simulink model "adas_acc_simulink"  (Simulink 8.8)
settings: Solver=FixedStepDiscrete  StartTime=0.0  StopTime=inf  RelTol=1e-3  EnableMultiTasking=on
libraries: SCANeR_API x7, simulink x3
settings Model: Creator=Administrateur  LastModifiedBy=gadam
settings OptimizationCC: ExpressionDepthLimit=2147483647  InitFltsAndDblsToZero=on  LifeSpan=1
settings DebuggingCC: SolverPrmCheckMsg=warning
settings SFSimCC: SimParseCustomCode=off
settings RTWCC: SystemTargetFile=ert_scanerapi.tlc  TemplateMakefile=ert_scanerapi_vc.tmf  Description=SCANeR API Real-Time Workshop Embedded Coder (no auto configuration)  TargetLang=C++
settings CodeAppCC: IgnoreCustomStorageClasses=off  CustomSymbolStrType=$N$R$M  InternalIdentifier=Classic
settings STFCustomTargetCC: ModelReferenceCompliant=off  CombineOutputUpdateFcns=on  ERTCustomFileBanners=on  RemoveResetFunc=on  MATLABClassNameForMDSCustomization=Simulink.SoftwareTarget.ERTCustomization  CPPClassGenCompliant=on  GRTInterface=off  SystemTargetFile=ert_scanerapi.tlc
settings ERTTargetCC: MultiwordLength=2048  ModelReferenceCompliant=off  ParMdlRefBuildCompliant=off  CompOptLevelCompliant=off  ConcurrentExecutionCompliant=off  ERTFirstTimeCompliant=off  SupportContinuousTime=on  SupportNonInlinedSFcns=on  ModelStepFunctionPrototypeControlCompliant=off  UseToolchainInfoCompliant=off  ExtModeMexFile=noextcomm  ERTCustomFileTemplate=example_file_process.tlc  ConvertIfToSwitch=off  SuppressUnreachableDefaultCases=off
settings CustomProperty: DataType=string  Value=M:\SCANER~1.4\APIs\simulink\SCANER~1

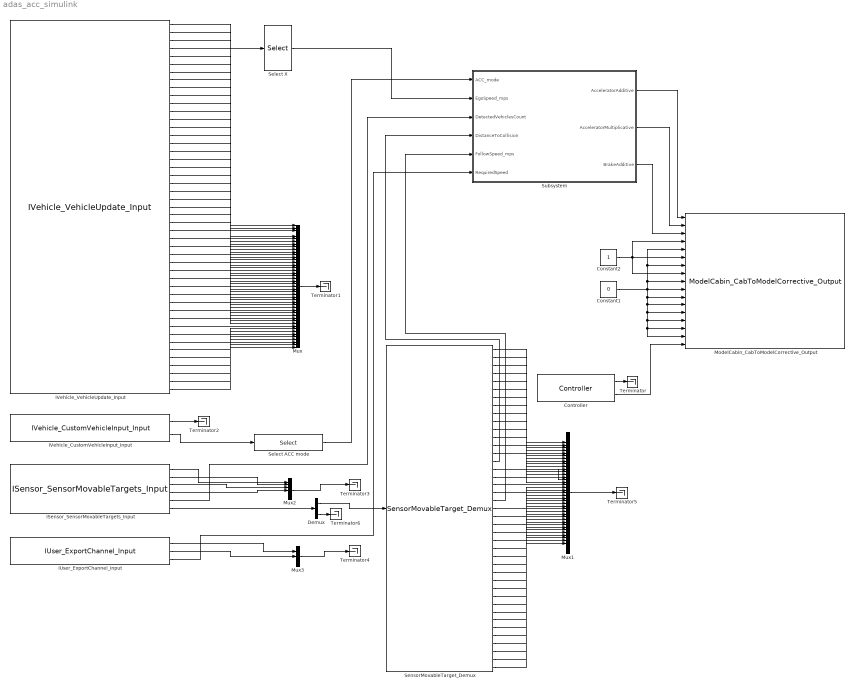
== system adas_acc_simulink ==
  Constant1 : Constant  Value=0
  Constant2 : Constant
  Controller : SCANeR_API/Controller  Config='DEMO_ADAS'  ProcName='SIMULINK_ACC'  Frequency=100  NetworkOutputFrequency=10  TimeOut=30  IsSynchronized=off
  Demux : Demux  Outputs=2
  ISensor_SensorMovableTargets_Input : SCANeR_API/Network inputs/ISensor/ISensor_SensorMovableTargets_Input  Priority=2  ev=off  globalId=300000
  IUser_ExportChannel_Input : SCANeR_API/Network inputs/IUser/IUser_ExportChannel_Input  Priority=2  ev=off  no=66
  IVehicle_CustomVehicleInput_Input : SCANeR_API/Network inputs/IVehicle/IVehicle_CustomVehicleInput_Input  Priority=2  ev=off  vhlId=0
  IVehicle_VehicleUpdate_Input : SCANeR_API/Network inputs/IVehicle/IVehicle_VehicleUpdate_Input  Priority=2  ev=off  vhlId=0
  ModelCabin_CabToModelCorrective_Output : SCANeR_API/SHM outputs/ModelCabin/ModelCabin_CabToModelCorrective_Output  Priority=2  shmId=0
  Mux : Mux  Inputs=47
  Mux1 : Mux  Inputs=39
  Mux2 : Mux  Inputs=6
  Mux3 : Mux  Inputs=3
  Select ACC mode : Selector  IndexMode=Zero-based  InputPortWidth=256  IndexOptions=Index vector (dialog)  Indices=2  OutputSizes=1
  Select X : Selector  IndexMode=Zero-based  InputPortWidth=6  IndexOptions=Index vector (dialog)  Indices=0  OutputSizes=1
  SensorMovableTarget_Demux : SCANeR_API/Structures/SensorMovableTarget_Demux
  Subsystem : Subsystem
  Terminator{,1..6} (7 alike) : Terminator
  wires:
  Controller/2 -> ModelCabin_CabToModelCorrective_Output/17
  Controller/1 -> Terminator/1
  Constant1/1 -> ModelCabin_CabToModelCorrective_Output/5, ModelCabin_CabToModelCorrective_Output/7, ModelCabin_CabToModelCorrective_Output/9, ModelCabin_CabToModelCorrective_Output/11, ModelCabin_CabToModelCorrective_Output/12, ModelCabin_CabToModelCorrective_Output/13, ModelCabin_CabToModelCorrective_Output/14, ModelCabin_CabToModelCorrective_Output/15, ModelCabin_CabToModelCorrective_Output/16, ModelCabin_CabToModelCorrective_Output/10
  Constant2/1 -> ModelCabin_CabToModelCorrective_Output/4, ModelCabin_CabToModelCorrective_Output/6, ModelCabin_CabToModelCorrective_Output/8
  IVehicle_VehicleUpdate_Input/39 -> Mux/39
  IVehicle_VehicleUpdate_Input/38 -> Mux/38
  IVehicle_VehicleUpdate_Input/40 -> Mux/40
  IVehicle_VehicleUpdate_Input/37 -> Mux/37
  IVehicle_VehicleUpdate_Input/41 -> Mux/41
  IVehicle_VehicleUpdate_Input/36 -> Mux/36
  IVehicle_VehicleUpdate_Input/42 -> Mux/42
  IVehicle_VehicleUpdate_Input/35 -> Mux/35
  IVehicle_VehicleUpdate_Input/43 -> Mux/43
  IVehicle_VehicleUpdate_Input/34 -> Mux/34
  IVehicle_VehicleUpdate_Input/44 -> Mux/44
  IVehicle_VehicleUpdate_Input/33 -> Mux/33
  IVehicle_VehicleUpdate_Input/45 -> Mux/45
  IVehicle_VehicleUpdate_Input/32 -> Mux/32
  IVehicle_VehicleUpdate_Input/46 -> Mux/46
  IVehicle_VehicleUpdate_Input/31 -> Mux/31
  IVehicle_VehicleUpdate_Input/47 -> Mux/47
  IVehicle_VehicleUpdate_Input/30 -> Mux/30
  IVehicle_VehicleUpdate_Input/29 -> Mux/29
  IVehicle_VehicleUpdate_Input/28 -> Mux/28
  IVehicle_VehicleUpdate_Input/27 -> Mux/27
  IVehicle_VehicleUpdate_Input/26 -> Mux/26
  IVehicle_VehicleUpdate_Input/25 -> Mux/25
  IVehicle_VehicleUpdate_Input/24 -> Mux/24
  IVehicle_VehicleUpdate_Input/23 -> Mux/23
  IVehicle_VehicleUpdate_Input/22 -> Mux/22
  IVehicle_VehicleUpdate_Input/21 -> Mux/21
  IVehicle_VehicleUpdate_Input/20 -> Mux/20
  IVehicle_VehicleUpdate_Input/19 -> Mux/19
  IVehicle_VehicleUpdate_Input/18 -> Mux/18
  IVehicle_VehicleUpdate_Input/17 -> Mux/17
  IVehicle_VehicleUpdate_Input/16 -> Mux/16
  IVehicle_VehicleUpdate_Input/15 -> Mux/15
  IVehicle_VehicleUpdate_Input/14 -> Mux/14
  IVehicle_VehicleUpdate_Input/13 -> Mux/13
  IVehicle_VehicleUpdate_Input/12 -> Mux/12
  IVehicle_VehicleUpdate_Input/11 -> Mux/11
  IVehicle_VehicleUpdate_Input/10 -> Mux/10
  IVehicle_VehicleUpdate_Input/9 -> Mux/9
  IVehicle_VehicleUpdate_Input/8 -> Mux/8
  IVehicle_VehicleUpdate_Input/7 -> Mux/7
  IVehicle_VehicleUpdate_Input/6 -> Mux/6
  IVehicle_VehicleUpdate_Input/5 -> Mux/5
  IVehicle_VehicleUpdate_Input/3 -> Mux/3
  IVehicle_VehicleUpdate_Input/2 -> Mux/2
  IVehicle_VehicleUpdate_Input/1 -> Mux/1
  ISensor_SensorMovableTargets_Input/3 -> Mux2/3
  ISensor_SensorMovableTargets_Input/4 -> Mux2/4
  ISensor_SensorMovableTargets_Input/2 -> Mux2/2
  ISensor_SensorMovableTargets_Input/1 -> Mux2/1
  IUser_ExportChannel_Input/2 -> Mux3/2
  IUser_ExportChannel_Input/1 -> Mux3/1
  Mux3/1 -> Terminator4/1
  Mux2/1 -> Terminator3/1
  Mux/1 -> Terminator1/1
  Subsystem/3(BrakeAdditive) -> ModelCabin_CabToModelCorrective_Output/3
  Subsystem/2(AcceleratorMultiplicative) -> ModelCabin_CabToModelCorrective_Output/2
  Subsystem/1(AcceleratorAdditive) -> ModelCabin_CabToModelCorrective_Output/1
  IVehicle_CustomVehicleInput_Input/1 -> Terminator2/1
  IVehicle_VehicleUpdate_Input/4 -> Select X/1
  Select X/1 -> Subsystem/2(EgoSpeed_mps)
  ISensor_SensorMovableTargets_Input/5 -> Subsystem/3(DetectedVehiclesCount)
  ISensor_SensorMovableTargets_Input/6 -> Demux/1
  Demux/1 -> SensorMovableTarget_Demux/1
  SensorMovableTarget_Demux/15 -> Subsystem/4(DistanceToCollision)
  SensorMovableTarget_Demux/20 -> Subsystem/5(FollowSpeed_mps)
  IUser_ExportChannel_Input/3 -> Subsystem/6(RequiredSpeed)
  SensorMovableTarget_Demux/16 -> Mux1/15
  SensorMovableTarget_Demux/17 -> Mux1/16
  SensorMovableTarget_Demux/18 -> Mux1/17
  SensorMovableTarget_Demux/14 -> Mux1/14
  SensorMovableTarget_Demux/19 -> Mux1/18
  SensorMovableTarget_Demux/13 -> Mux1/13
  SensorMovableTarget_Demux/12 -> Mux1/12
  SensorMovableTarget_Demux/11 -> Mux1/11
  SensorMovableTarget_Demux/21 -> Mux1/19
  SensorMovableTarget_Demux/10 -> Mux1/10
  SensorMovableTarget_Demux/22 -> Mux1/20
  SensorMovableTarget_Demux/9 -> Mux1/9
  SensorMovableTarget_Demux/23 -> Mux1/21
  SensorMovableTarget_Demux/8 -> Mux1/8
  SensorMovableTarget_Demux/24 -> Mux1/22
  SensorMovableTarget_Demux/7 -> Mux1/7
  SensorMovableTarget_Demux/25 -> Mux1/23
  SensorMovableTarget_Demux/6 -> Mux1/6
  SensorMovableTarget_Demux/26 -> Mux1/24
  SensorMovableTarget_Demux/5 -> Mux1/5
  SensorMovableTarget_Demux/27 -> Mux1/25
  SensorMovableTarget_Demux/4 -> Mux1/4
  SensorMovableTarget_Demux/28 -> Mux1/26
  SensorMovableTarget_Demux/3 -> Mux1/3
  SensorMovableTarget_Demux/29 -> Mux1/27
  SensorMovableTarget_Demux/2 -> Mux1/2
  SensorMovableTarget_Demux/30 -> Mux1/28
  SensorMovableTarget_Demux/1 -> Mux1/1
  SensorMovableTarget_Demux/31 -> Mux1/29
  SensorMovableTarget_Demux/32 -> Mux1/30
  SensorMovableTarget_Demux/33 -> Mux1/31
  SensorMovableTarget_Demux/34 -> Mux1/32
  SensorMovableTarget_Demux/35 -> Mux1/33
  SensorMovableTarget_Demux/36 -> Mux1/34
  SensorMovableTarget_Demux/37 -> Mux1/35
  SensorMovableTarget_Demux/38 -> Mux1/36
  SensorMovableTarget_Demux/39 -> Mux1/37
  SensorMovableTarget_Demux/40 -> Mux1/38
  SensorMovableTarget_Demux/41 -> Mux1/39
  Mux1/1 -> Terminator5/1
  Demux/2 -> Terminator6/1
  Select ACC mode/1 -> Subsystem/1(ACC_mode)
  IVehicle_CustomVehicleInput_Input/2 -> Select ACC mode/1

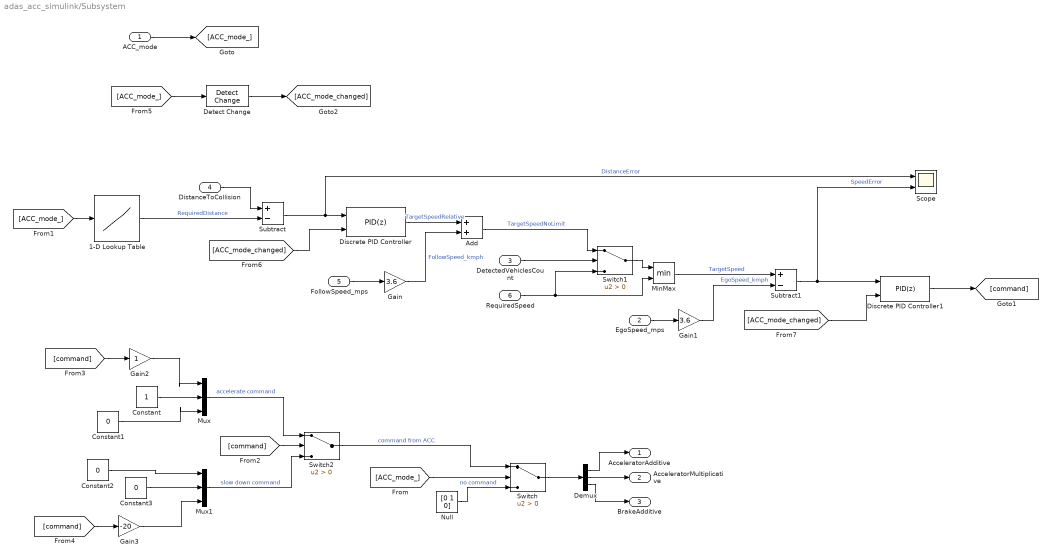
== system adas_acc_simulink/Subsystem ==
  ACC_mode : Inport
  EgoSpeed_mps : Inport  Port=2
  DetectedVehiclesCount : Inport  Port=3
  DistanceToCollision : Inport  Port=4
  FollowSpeed_mps : Inport  Port=5
  RequiredSpeed : Inport  Port=6
  1-D Lookup Table : Lookup_n-D  NumberOfTableDimensions=1  BreakpointsSpecification=Even spacing  BreakpointsForDimension1=[1,2,3,4]  Table=[20,30,40,50]  InternalRulePriority=Speed  RndMeth=Simplest  InputSameDT=on
  Add : Sum
  Constant : Constant
  Constant1 : Constant  Value=0
  Constant2 : Constant  Value=0
  Constant3 : Constant  Value=0
  Demux : Demux  Outputs=3
  Detect Change : simulink/Logic and Bit Operations/Detect Change  vinit=0  OutDataTypeStr=boolean
  Discrete PID Controller : simulink/Continuous/PID Controller  Controller=PID  TimeDomain=Discrete-time  SampleTime=-1  IntegratorMethod=Forward Euler  FilterMethod=Forward Euler  Form=Parallel  UseFilter=on  ControllerParametersSource=internal  P=0.5  I=1e-4  D=0.5  N=100  InitialConditionSource=internal  InitialConditionForIntegrator=0  InitialConditionForFilter=0  ExternalReset=rising  LimitOutput=on  UpperSaturationLimit=200  LowerSaturationLimit=0  LinearizeAsGain=off  AntiWindupMode=none  Kb=1  TrackingMode=off  Kt=1  PParamMin=[]  PParamMax=[]  IParamMin=[]  IParamMax=[]  DParamMin=[]  DParamMax=[]  NParamMin=[]  NParamMax=[]  KbParamMin=[]  KbParamMax=[]  KtParamMin=[]  KtParamMax=[]  POutMin=[]  POutMax=[]  IOutMin=[]  IOutMax=[]  DOutMin=[]  DOutMax=[]  NOutMin=[]  NOutMax=[]  KbOutMin=[]  KbOutMax=[]  KtOutMin=[]  KtOutMax=[]  IntegratorOutMin=[]  IntegratorOutMax=[]  FilterOutMin=[]  FilterOutMax=[]  SumOutMin=[]  SumOutMax=[]  SumI1OutMin=[]  SumI1OutMax=[]  SumI2OutMin=[]  SumI2OutMax=[]  SumI3OutMin=[]  SumI3OutMax=[]  SumDOutMin=[]  SumDOutMax=[]  SaturationOutMin=[]  SaturationOutMax=[]  IntegratorContinuousStateAttributes=''  IntegratorStateMustResolveToSignalObject=off  IntegratorRTWStateStorageClass=Auto  FilterContinuousStateAttributes=''  FilterStateMustResolveToSignalObject=off  FilterRTWStateStorageClass=Auto  DifferentiatorICPrevScaledInput=0  DifferentiatorOutMin=[]  DifferentiatorOutMax=[]
  Discrete PID Controller1 : simulink/Continuous/PID Controller  Controller=PID  TimeDomain=Discrete-time  SampleTime=-1  IntegratorMethod=Forward Euler  FilterMethod=Forward Euler  Form=Parallel  UseFilter=on  ControllerParametersSource=internal  P=0.1  I=5e-4  D=0.1  N=100  InitialConditionSource=internal  InitialConditionForIntegrator=0  InitialConditionForFilter=0  ExternalReset=rising  LimitOutput=on  UpperSaturationLimit=1  LowerSaturationLimit=-1  LinearizeAsGain=off  AntiWindupMode=none  Kb=1  TrackingMode=off  Kt=1  PParamMin=[]  PParamMax=[]  IParamMin=[]  IParamMax=[]  DParamMin=[]  DParamMax=[]  NParamMin=[]  NParamMax=[]  KbParamMin=[]  KbParamMax=[]  KtParamMin=[]  KtParamMax=[]  POutMin=[]  POutMax=[]  IOutMin=[]  IOutMax=[]  DOutMin=[]  DOutMax=[]  NOutMin=[]  NOutMax=[]  KbOutMin=[]  KbOutMax=[]  KtOutMin=[]  KtOutMax=[]  IntegratorOutMin=[]  IntegratorOutMax=[]  FilterOutMin=[]  FilterOutMax=[]  SumOutMin=[]  SumOutMax=[]  SumI1OutMin=[]  SumI1OutMax=[]  SumI2OutMin=[]  SumI2OutMax=[]  SumI3OutMin=[]  SumI3OutMax=[]  SumDOutMin=[]  SumDOutMax=[]  SaturationOutMin=[]  SaturationOutMax=[]  IntegratorContinuousStateAttributes=''  IntegratorStateMustResolveToSignalObject=off  IntegratorRTWStateStorageClass=Auto  FilterContinuousStateAttributes=''  FilterStateMustResolveToSignalObject=off  FilterRTWStateStorageClass=Auto  DifferentiatorICPrevScaledInput=0  DifferentiatorOutMin=[]  DifferentiatorOutMax=[]
  Gain : Gain  Gain=3.6
  Gain1 : Gain  Gain=3.6
  Gain2 : Gain
  Gain3 : Gain  Gain=-20
  MinMax : MinMax  Inputs=2
  Mux : Mux  Inputs=3
  Mux1 : Mux  Inputs=3
  Null : Constant  Value=[0 1 0]
  Scope : Scope  NumInputPorts=2
  Subtract : Sum  Inputs=+-
  Subtract1 : Sum  Inputs=+-
  Switch : Switch  Criteria=u2 > Threshold
  Switch1 : Switch  Criteria=u2 > Threshold
  Switch2 : Switch  Criteria=u2 > Threshold
  AcceleratorAdditive : Outport
  AcceleratorMultiplicative : Outport  Port=2
  BrakeAdditive : Outport  Port=3
  wires:
  Demux/1 -> AcceleratorAdditive/1
  Demux/2 -> AcceleratorMultiplicative/1
  Demux/3 -> BrakeAdditive/1
  Switch/1 -> Demux/1
  Null/1 -> Switch/3  "no command"
  DistanceToCollision/1 -> Subtract/1
  DetectedVehiclesCount/1 -> Switch1/2
  FollowSpeed_mps/1 -> Gain/1
  Gain/1 -> Add/2  "FollowSpeed_kmph"
  Subtract/1 -> Scope/1, Discrete PID Controller/1  "DistanceError"
  Add/1 -> Switch1/1  "TargetSpeedNoLimit"
  RequiredSpeed/1 -> MinMax/2, Switch1/3
  1-D Lookup Table/1 -> Subtract/2  "RequiredDistance"
  ACC_mode/1 -> [ACC_mode_]
  [ACC_mode_] -> 1-D Lookup Table/1
  [ACC_mode_] -> Switch/2
  EgoSpeed_mps/1 -> Gain1/1
  Gain1/1 -> Subtract1/2  "EgoSpeed_kmph"
  Subtract1/1 -> Scope/2, Discrete PID Controller1/1  "SpeedError"
  [command] -> Switch2/2
  Mux1/1 -> Switch2/3  "slow down command"
  Mux/1 -> Switch2/1  "accelerate command"
  Constant3/1 -> Mux1/2
  Constant2/1 -> Mux1/1
  Constant/1 -> Mux/2
  Constant1/1 -> Mux/3
  [command] -> Gain2/1
  Gain2/1 -> Mux/1
  [command] -> Gain3/1
  Gain3/1 -> Mux1/3
  Switch2/1 -> Switch/1  "command from ACC"
  Discrete PID Controller/1 -> Add/1  "TargetSpeedRelative"
  MinMax/1 -> Subtract1/1  "TargetSpeed"
  Switch1/1 -> MinMax/1
  [ACC_mode_] -> Detect Change/1
  Detect Change/1 -> [ACC_mode_changed]
  [ACC_mode_changed] -> Discrete PID Controller/2
  [ACC_mode_changed] -> Discrete PID Controller1/2
  Discrete PID Controller1/1 -> [command]
